simulink model "IMPLICIT_2ODE_EX4_sim"  (Simulink 10.0)
settings: Solver=daessc  StartTime=0.0  StopTime=13  RelTol=1e-3
settings Model: Creator=sulaymon.eshkabilov  LastModifiedBy=sulaymon.eshkabilov
settings DataIOCC: SaveFormat=Dataset  ReturnWorkspaceOutputs=on
settings OptimizationCC: LifeSpan=auto
settings DebuggingCC: UnderspecifiedInitializationDetection=Simplified  MergeDetectMultiDrivingBlocksExec=error  SFUnexpectedBacktrackingDiag=error  SFNoUnconditionalDefaultTransitionDiag=error  SFExecutionAtInitializationDiag=warning  ArithmeticOperatorsInVariantConditions=error
settings HardwareCC: ProdBitPerPointer=64  ProdBitPerSizeT=64  ProdBitPerPtrDiffT=64  ProdLargestAtomicFloat=Float  ProdIntDivRoundTo=Zero  ProdEndianess=LittleEndian  ProdWordSize=64  ProdHWDeviceType=Intel->x86-64 (Windows64)
settings ModelReferenceCC: PropagateSignalLabelsOutOfModel=on
settings SFSimCC: SimUseLocalCustomCode=on  CustomCodeUndefinedFunction=FilterOut
settings RTWCC: RTWUseLocalCustomCode=on
settings CodeAppCC: StateflowObjectComments=off
settings GRTTargetCC: TargetLangStandard=C99 (ISO)  CombineOutputUpdateFcns=on  GRTInterface=off
settings ConfigComp: CovMetricSettings=dwe  CovHtmlReporting=off  CovSaveCumulativeToWorkspaceVar=off  CovSaveSingleToWorkspaceVar=off

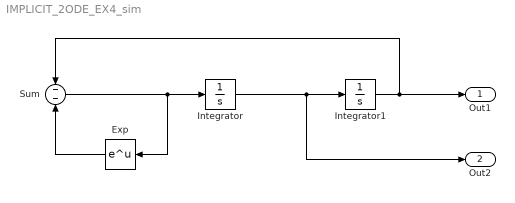
== system IMPLICIT_2ODE_EX4_sim ==
  Exp : Math  SignedPower=off  SaturateOnIntegerOverflow=on
  Integrator : Integrator
  Integrator1 : Integrator  InitialCondition=1
  Sum : Sum  Inputs=--
  Out1 : Outport
  Out2 : Outport  Port=2
  wires:
  Integrator/1 -> Out2/1, Integrator1/1
  Sum/1 -> Exp/1, Integrator/1
  Exp/1 -> Sum/2
  Integrator1/1 -> Out1/1, Sum/1
